simulink model "CDMA_test"  (Simulink 7.7)
settings: Solver=FixedStepDiscrete  StartTime=0.0  StopTime=10  RelTol=1e-3
libraries: commrandsrc2 x6
settings Model: Creator=ArunKB  LastModifiedBy=ArunKB

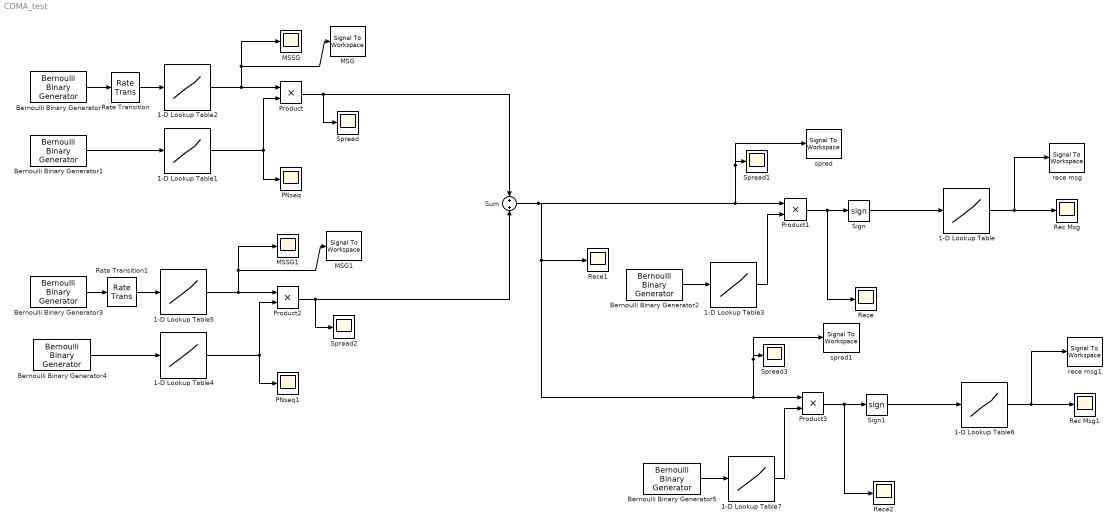
== system CDMA_test ==
  1-D Lookup Table : Lookup_n-D  NumberOfTableDimensions=1  BreakpointsForDimension1=[-1,0,1]  Table=[-1,-1,1]  RndMeth=Simplest  InputSameDT=on
  1-D Lookup Table{1..5,7} (6 alike) : Lookup_n-D  NumberOfTableDimensions=1  BreakpointsForDimension1=[0 1]  Table=[-1 1]  RndMeth=Simplest  InputSameDT=on
  1-D Lookup Table6 : Lookup_n-D  NumberOfTableDimensions=1  BreakpointsForDimension1=[-1,0,1]  Table=[-1,-1,1]  RndMeth=Simplest  InputSameDT=on
  Bernoulli Binary Generator : commrandsrc2/Bernoulli Binary Generator  SystemSampleTime=-1  P=0.5  seed=randseed  Ts=1  frameBased=off  sampPerFrame=1  orient=off  outDataType=double
  Bernoulli Binary Generator1 : commrandsrc2/Bernoulli Binary Generator  SystemSampleTime=-1  P=0.5  seed=88  Ts=.01  frameBased=off  sampPerFrame=1  orient=off  outDataType=double
  Bernoulli Binary Generator2 : commrandsrc2/Bernoulli Binary Generator  SystemSampleTime=-1  P=0.5  seed=45  Ts=.01  frameBased=off  sampPerFrame=1  orient=off  outDataType=double
  Bernoulli Binary Generator3 : commrandsrc2/Bernoulli Binary Generator  SystemSampleTime=-1  P=0.5  seed=randseed  Ts=1  frameBased=off  sampPerFrame=1  orient=off  outDataType=double
  Bernoulli Binary Generator4 : commrandsrc2/Bernoulli Binary Generator  SystemSampleTime=-1  P=0.5  seed=45  Ts=.01  frameBased=off  sampPerFrame=1  orient=off  outDataType=double
  Bernoulli Binary Generator5 : commrandsrc2/Bernoulli Binary Generator  SystemSampleTime=-1  P=0.5  seed=88  Ts=.01  frameBased=off  sampPerFrame=1  orient=off  outDataType=double
  MSG : SignalToWorkspace  VariableName=msg  SaveFormat=Array  Save2DMode=2-D array (concatenate along first dimension)
      settings: CopyFcn=dspblkcopystw(gcbh);
  MSG1 : SignalToWorkspace  VariableName=msg1  SaveFormat=Array  Save2DMode=2-D array (concatenate along first dimension)
      settings: CopyFcn=dspblkcopystw(gcbh);
  MSSG : Scope
  MSSG1 : Scope
      settings: SaveName=ScopeData6
  PNseq : Scope
      settings: SaveName=ScopeData2
  PNseq1 : Scope
      settings: SaveName=ScopeData7
  Product{,1..3} (4 alike) : Product  RndMeth=Zero
  Rate Transition : RateTransition
  Rate Transition1 : RateTransition
  Rec Msg : Scope
      settings: SaveName=ScopeData4
  Rec Msg1 : Scope
      settings: SaveName=ScopeData10
  Rece : Scope
      settings: SaveName=ScopeData3
  Rece1 : Scope
      settings: SaveName=ScopeData9
  Rece2 : Scope
      settings: SaveName=ScopeData11
  Sign : Signum
  Sign1 : Signum
  Spread{,1..3} (4 alike) : Scope
      Spread1 settings: SaveName=ScopeData5
      Spread2 settings: SaveName=ScopeData8
      Spread3 settings: SaveName=ScopeData12
  Sum : Sum  Inputs=+|+
  rece msg : SignalToWorkspace  VariableName=rece  SaveFormat=Array  Save2DMode=2-D array (concatenate along first dimension)
      settings: CopyFcn=dspblkcopystw(gcbh);
  rece msg1 : SignalToWorkspace  VariableName=rece1  SaveFormat=Array  Save2DMode=2-D array (concatenate along first dimension)
      settings: CopyFcn=dspblkcopystw(gcbh);
  spred : SignalToWorkspace  VariableName=spread  SaveFormat=Array  Save2DMode=2-D array (concatenate along first dimension)
      settings: CopyFcn=dspblkcopystw(gcbh);
  spred1 : SignalToWorkspace  VariableName=spread1  SaveFormat=Array  Save2DMode=2-D array (concatenate along first dimension)
      settings: CopyFcn=dspblkcopystw(gcbh);
  wires:
  1-D Lookup Table2/1 -> Product/1, MSSG/1, MSG/1
  Rate Transition/1 -> 1-D Lookup Table2/1
  1-D Lookup Table1/1 -> Product/2, PNseq/1
  Bernoulli Binary Generator/1 -> Rate Transition/1
  1-D Lookup Table3/1 -> Product1/2
  Product1/1 -> Rece/1, Sign/1
  1-D Lookup Table/1 -> rece msg/1, Rec Msg/1
  Sign/1 -> 1-D Lookup Table/1
  1-D Lookup Table5/1 -> MSG1/1, MSSG1/1, Product2/1
  Rate Transition1/1 -> 1-D Lookup Table5/1
  1-D Lookup Table4/1 -> PNseq1/1, Product2/2
  Bernoulli Binary Generator3/1 -> Rate Transition1/1
  Sum/1 -> Product1/1, Spread1/1, spred/1, Rece1/1, spred1/1, Spread3/1, Product3/1
  Bernoulli Binary Generator4/1 -> 1-D Lookup Table4/1
  Bernoulli Binary Generator1/1 -> 1-D Lookup Table1/1
  Product/1 -> Sum/1, Spread/1
  Product2/1 -> Sum/2, Spread2/1
  Bernoulli Binary Generator2/1 -> 1-D Lookup Table3/1
  1-D Lookup Table7/1 -> Product3/2
  Product3/1 -> Sign1/1, Rece2/1
  1-D Lookup Table6/1 -> Rec Msg1/1, rece msg1/1
  Sign1/1 -> 1-D Lookup Table6/1
  Bernoulli Binary Generator5/1 -> 1-D Lookup Table7/1
